simulink model "Direct_form"  (R2020b)
settings: Solver=VariableStepAuto  StartTime=0.0  StopTime=10.0  RelTol=1e-3
settings Model: Creator=Shivashis  LastModifiedBy=Shivashis
settings DataIOCC: SaveOutput=off  SaveTime=off

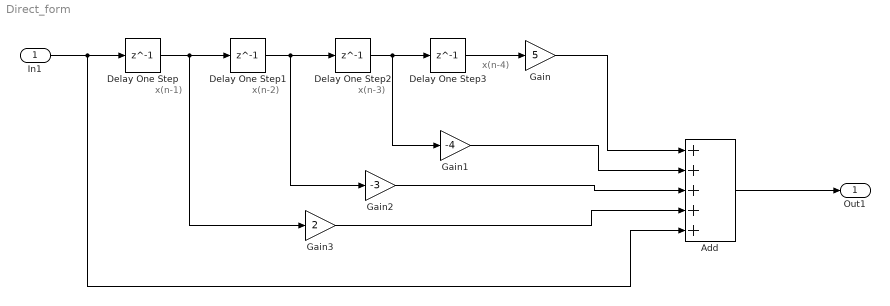
== system Direct_form ==
  note: x(n-2)
  note: x(n-3)
  note: x(n-1)
  note: x(n-4)
  In1 : Inport  OutDataTypeStr=double  PortDimensions=1  SampleTime=0
  Add : Sum  Inputs=+++++
  Delay One Step{,1..3} (4 alike) : Delay  DelayLength=1
  Gain : Gain  Gain=5
  Gain1 : Gain  Gain=-4
  Gain2 : Gain  Gain=-3
  Gain3 : Gain  Gain=2
  Out1 : Outport  OutDataTypeStr=double  PortDimensions=1  SampleTime=0
  wires:
  Delay One Step3/1 -> Gain/1
  Gain3/1 -> Add/4
  Gain/1 -> Add/1
  Gain2/1 -> Add/3
  Delay One Step2/1 -> Delay One Step3/1, Gain1/1
  Delay One Step/1 -> Delay One Step1/1, Gain3/1
  In1/1 -> Delay One Step/1, Add/5
  Gain1/1 -> Add/2
  Delay One Step1/1 -> Delay One Step2/1, Gain2/1
  Add/1 -> Out1/1
